simulink library "BEML_EMU_BrakesInput_Lib"  (R2019b)
settings: Solver=VariableStepAuto  StartTime=0.0  StopTime=10.0  RelTol=1e-3
undefined symbols (not defined in the file): BrakeCylinderPressure, BrakesSampleTime, ElectricParkBrakeApplication, FrictionBrakeForceVariation, ManualHandBrakeApplication, ParkBrakeOverride, ParkBrakePressure, VehicleVelocity, WheelSpeed
settings Model: Creator=rleighton  LastModifiedBy=hinganes
settings DebuggingCC: ArithmeticOperatorsInVariantConditions=warning
settings SFSimCC: SimUseLocalCustomCode=off  CustomCodeUndefinedFunction=UseInterfaceOnly
settings RTWCC: RTWUseLocalCustomCode=off

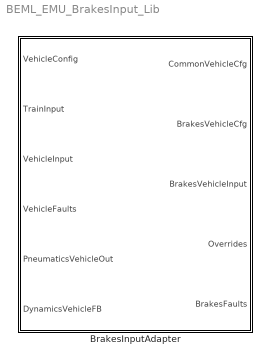
== system BEML_EMU_BrakesInput_Lib ==
  BrakesInputAdapter : Subsystem  TreatAsAtomicUnit=on  SystemSampleTime=BrakesSampleTime

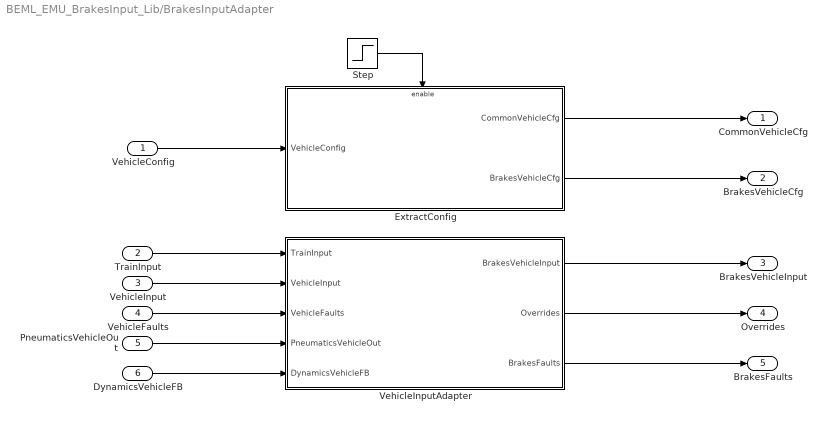
== system BEML_EMU_BrakesInput_Lib/BrakesInputAdapter ==
  VehicleConfig : Inport
  TrainInput : Inport  Port=2
  VehicleInput : Inport  Port=3
  VehicleFaults : Inport  Port=4
  PneumaticsVehicleOut : Inport  Port=5
  DynamicsVehicleFB : Inport  Port=6
  ExtractConfig : Subsystem
  Step : Step  Before=1  After=0
  VehicleInputAdapter : Subsystem
  CommonVehicleCfg : Outport  VectorParamsAs1DForOutWhenUnconnected=off
  BrakesVehicleCfg : Outport  Port=2  VectorParamsAs1DForOutWhenUnconnected=off
  BrakesVehicleInput : Outport  Port=3  VectorParamsAs1DForOutWhenUnconnected=off
  Overrides : Outport  Port=4  VectorParamsAs1DForOutWhenUnconnected=off
  BrakesFaults : Outport  Port=5  VectorParamsAs1DForOutWhenUnconnected=off
  wires:
  TrainInput/1 -> VehicleInputAdapter/1(TrainInput)
  VehicleInput/1 -> VehicleInputAdapter/2(VehicleInput)
  PneumaticsVehicleOut/1 -> VehicleInputAdapter/4(PneumaticsVehicleOut)
  DynamicsVehicleFB/1 -> VehicleInputAdapter/5(DynamicsVehicleFB)
  VehicleConfig/1 -> ExtractConfig/1(VehicleConfig)
  ExtractConfig/1(CommonVehicleCfg) -> CommonVehicleCfg/1
  ExtractConfig/2(BrakesVehicleCfg) -> BrakesVehicleCfg/1
  Step/1 -> ExtractConfig/Enable
  VehicleFaults/1 -> VehicleInputAdapter/3(VehicleFaults)
  VehicleInputAdapter/1(BrakesVehicleInput) -> BrakesVehicleInput/1
  VehicleInputAdapter/2(Overrides) -> Overrides/1
  VehicleInputAdapter/3(BrakesFaults) -> BrakesFaults/1

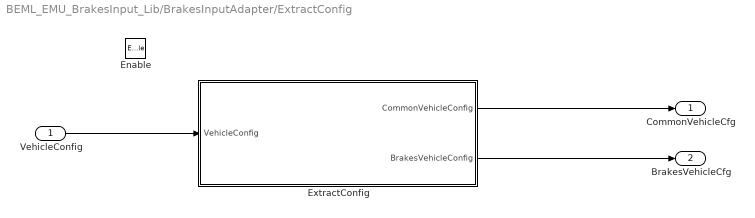
== system BEML_EMU_BrakesInput_Lib/BrakesInputAdapter/ExtractConfig ==
  VehicleConfig : Inport
  Enable : EnablePort
  ExtractConfig : Subsystem
  CommonVehicleCfg : Outport  VectorParamsAs1DForOutWhenUnconnected=off
  BrakesVehicleCfg : Outport  Port=2  VectorParamsAs1DForOutWhenUnconnected=off
  wires:
  ExtractConfig/2(BrakesVehicleConfig) -> BrakesVehicleCfg/1
  ExtractConfig/1(CommonVehicleConfig) -> CommonVehicleCfg/1
  VehicleConfig/1 -> ExtractConfig/1(VehicleConfig)

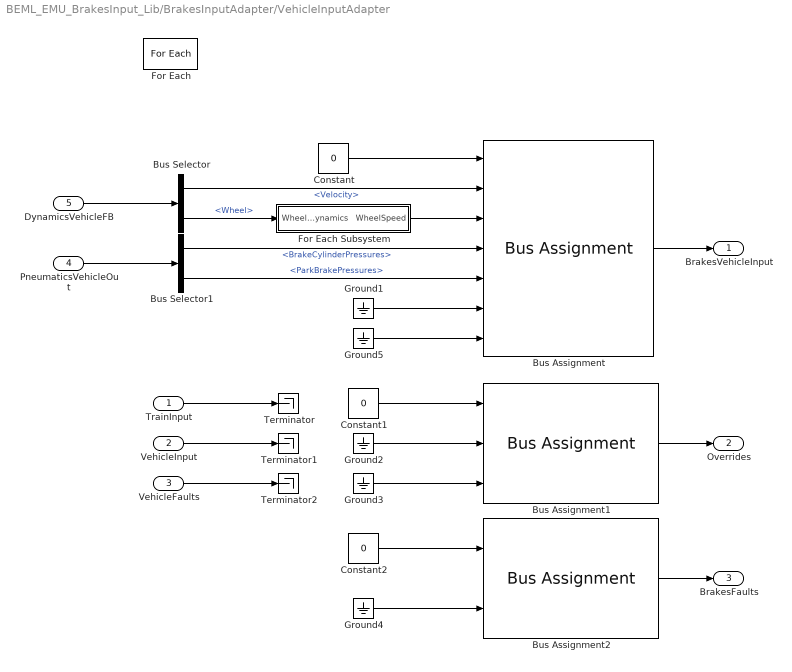
== system BEML_EMU_BrakesInput_Lib/BrakesInputAdapter/VehicleInputAdapter ==
  TrainInput : Inport
  VehicleInput : Inport  Port=2  Partition=on  PartitionDimension=1  PartitionWidth=1  PartitionOffset=0
  VehicleFaults : Inport  Port=3  Partition=on  PartitionDimension=1  PartitionWidth=1  PartitionOffset=0
  PneumaticsVehicleOut : Inport  Port=4  Partition=on  PartitionDimension=1  PartitionWidth=1  PartitionOffset=0
  DynamicsVehicleFB : Inport  Port=5  Partition=on  PartitionDimension=1  PartitionWidth=1  PartitionOffset=0
  Bus Assignment : BusAssignment  AssignedSignals=VehicleVelocity,WheelSpeed,BrakeCylinderPressure,ParkBrakePressure,ManualHandBrakeApplication,ElectricParkBrakeApplication
  Bus Assignment1 : BusAssignment  AssignedSignals=FrictionBrakeForceVariation,ParkBrakeOverride
  Bus Assignment2 : BusAssignment  AssignedSignals=BrakeShoeOverheatFault
  Bus Selector : BusSelector  OutputSignals=Inertia.Velocity,Wheel
  Bus Selector1 : BusSelector  OutputSignals=AxleBrakes.BrakeCylinderPressures,AxleBrakes.ParkBrakePressures
  Constant : Constant  Value=0  OutDataTypeStr=Bus: BD_TrainBrakes_In_Vehicle
  Constant1 : Constant  Value=0  OutDataTypeStr=Bus: BD_TrainBrakes_In_Vehicle_Overrides
  Constant2 : Constant  Value=0  OutDataTypeStr=Bus: BD_TrainBrakes_In_Vehicle_Faults
  For Each : ForEach  DisableCoverage=on
  For Each Subsystem : Subsystem  TreatAsAtomicUnit=on
  Ground{1..5} (5 alike) : Ground
  Terminator : Terminator
  Terminator1 : Terminator
  Terminator2 : Terminator
  BrakesVehicleInput : Outport  ConcatenationDimension=1  VectorParamsAs1DForOutWhenUnconnected=off
  Overrides : Outport  Port=2  ConcatenationDimension=1  VectorParamsAs1DForOutWhenUnconnected=off
  BrakesFaults : Outport  Port=3  ConcatenationDimension=1  VectorParamsAs1DForOutWhenUnconnected=off
  wires:
  Bus Selector1/2 -> Bus Assignment/5  "<ParkBrakePressures>"
  Bus Selector1/1 -> Bus Assignment/4  "<BrakeCylinderPressures>"
  For Each Subsystem/1(WheelSpeed) -> Bus Assignment/3
  Bus Selector/2 -> For Each Subsystem/1(WheelDynamics)  "<Wheel>"
  Bus Selector/1 -> Bus Assignment/2  "<Velocity>"
  Ground1/1 -> Bus Assignment/6
  Ground5/1 -> Bus Assignment/7
  TrainInput/1 -> Terminator/1
  VehicleInput/1 -> Terminator1/1
  VehicleFaults/1 -> Terminator2/1
  PneumaticsVehicleOut/1 -> Bus Selector1/1
  DynamicsVehicleFB/1 -> Bus Selector/1
  Constant/1 -> Bus Assignment/1
  Bus Assignment/1 -> BrakesVehicleInput/1
  Constant1/1 -> Bus Assignment1/1
  Ground3/1 -> Bus Assignment1/3
  Ground2/1 -> Bus Assignment1/2
  Bus Assignment1/1 -> Overrides/1
  Ground4/1 -> Bus Assignment2/2
  Constant2/1 -> Bus Assignment2/1
  Bus Assignment2/1 -> BrakesFaults/1

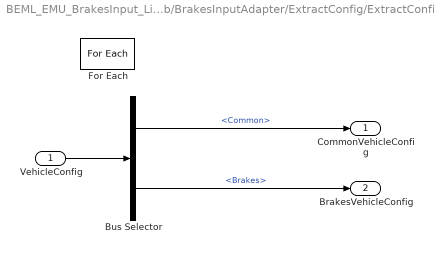
== system BEML_EMU_BrakesInput_Lib/BrakesInputAdapter/ExtractConfig/ExtractConfig ==
  VehicleConfig : Inport  Partition=on  PartitionDimension=1  PartitionWidth=1  PartitionOffset=0  BusOutputAsStruct=on
  Bus Selector : BusSelector  OutputSignals=Common,Brakes
  For Each : ForEach  DisableCoverage=on
  CommonVehicleConfig : Outport  ConcatenationDimension=1  VectorParamsAs1DForOutWhenUnconnected=off
  BrakesVehicleConfig : Outport  Port=2  ConcatenationDimension=1  VectorParamsAs1DForOutWhenUnconnected=off
  wires:
  VehicleConfig/1 -> Bus Selector/1
  Bus Selector/1 -> CommonVehicleConfig/1  "<Common>"
  Bus Selector/2 -> BrakesVehicleConfig/1  "<Brakes>"

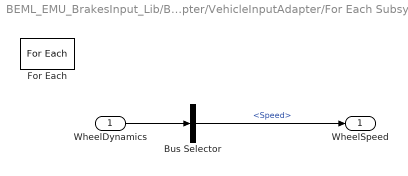
== system BEML_EMU_BrakesInput_Lib/BrakesInputAdapter/VehicleInputAdapter/For Each Subsystem ==
  WheelDynamics : Inport  Partition=on  PartitionDimension=1  PartitionWidth=1  PartitionOffset=0
  Bus Selector : BusSelector  OutputSignals=Speed
  For Each : ForEach  DisableCoverage=on
  WheelSpeed : Outport  ConcatenationDimension=1
  wires:
  Bus Selector/1 -> WheelSpeed/1  "<Speed>"
  WheelDynamics/1 -> Bus Selector/1
